simulink model "Log_Optitrack_TruckLab_A1"  (R2025b)
settings: Solver=ode4  StartTime=0  StopTime=130  FixedStep=1/120  RelTol=1e-3
undefined symbols (not defined in the file or in its folder): getRigidBodyPose
libraries: simulink_extras x2
settings Model: Creator=20212285  LastModifiedBy=20224886
settings SolverCC: AlgebraicLoopSolver=LineSearch
settings DataIOCC: ReturnWorkspaceOutputsName=s
settings OptimizationCC: EnhancedBackFolding=on  PassReuseOutputArgsAs=Individual arguments  ZeroExternalMemoryAtStartup=off  ZeroInternalMemoryAtStartup=off  MaxStackSize=64  OptimizeBlockOrder=speed  DifferentSizesBufferReuse=on  OptimizationCustomize=off  EfficientTunableParamExpr=on
settings DebuggingCC: ParameterTunabilityLossMsg=error  UnconnectedInputMsg=warning  UnconnectedOutputMsg=warning  UnconnectedLineMsg=warning
settings ModelReferenceCC: EnableRefExpFcnMdlSchedulingChecks=on
settings SFSimCC: MATLABDynamicMemAlloc=off  SimTargetLang=C++  SimDLTargetLibrary=mkl-dnn
settings RTWCC: SystemTargetFile=ert.tlc  HardwareBoard=Robot Operating System 2 (ROS 2)  TLCOptions="-aInlineSetEventsForThisBaseRateFcn=TLC_FALSE -aSuppressMultiTaskScheduler=TLC_FALSE  -aRateBasedStepFcn=0"  TemplateMakefile=ert_default_tmf  Toolchain=Colcon Tools  TargetLang=C++  GPUComputeCapability=3.5  Description=Embedded Coder
settings CodeAppCC: ForceParamTrailComments=on  IgnoreCustomStorageClasses=off  OperatorAnnotations=on  SimulinkDataObjDesc=on  SFDataObjDesc=on  InsertBlockDesc=on
settings ERTTargetCC: ExtModeTransport=2.0  ExtModeStaticAlloc=on  ExtModeAutomaticAllocSize=off  ExtModeMexFile=ext_xcp  ExtModeIntrfLevel=Level2 - Open  InlinedParameterPlacement=Hierarchical  RootIOFormat=Structure reference  DynamicArrayContainerType=coder::array  CodeInterfacePackaging=C++ class

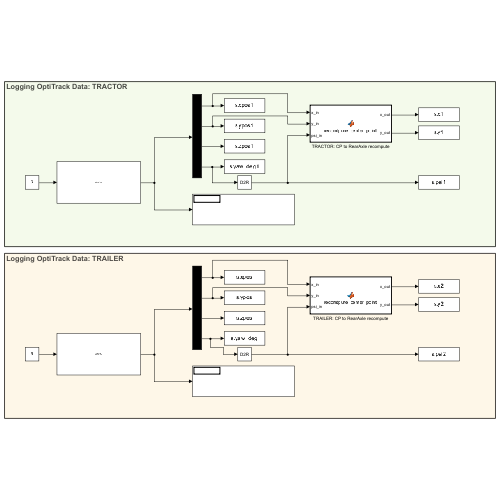
[thumbnail: Simulink's stored preview of the top-level diagram]
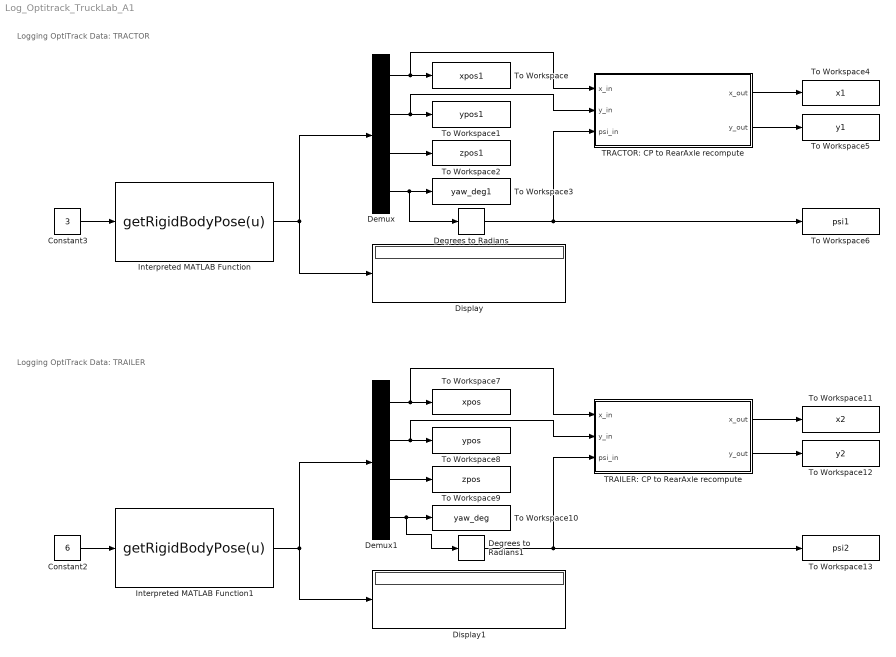
== system Log_Optitrack_TruckLab_A1 ==
  note: Logging OptiTrack Data: TRACTOR
  note: Logging OptiTrack Data: TRAILER
  Constant2 : Constant  Value=6
  Constant3 : Constant  Value=3
  Degrees to Radians : simulink_extras/Transformations/Degrees to Radians
  Degrees to Radians1 : simulink_extras/Transformations/Degrees to Radians
  Demux : Demux
  Demux1 : Demux
  Display : Display
  Display1 : Display
  Interpreted MATLAB Function : MATLABFcn  MATLABFcn=getRigidBodyPose(u)
  Interpreted MATLAB Function1 : MATLABFcn  MATLABFcn=getRigidBodyPose(u)
  TRACTOR: CP to RearAxle recompute : MATLAB Function  TreatAsAtomicUnit=on
  TRAILER: CP to RearAxle recompute : MATLAB Function  TreatAsAtomicUnit=on
  To Workspace : ToWorkspace  VariableName=xpos1  SaveFormat=Timeseries  SampleTime=-1
  To Workspace1 : ToWorkspace  VariableName=ypos1  SaveFormat=Timeseries  SampleTime=-1
  To Workspace10 : ToWorkspace  VariableName=yaw_deg  SaveFormat=Timeseries  SampleTime=-1
  To Workspace11 : ToWorkspace  VariableName=x2  SaveFormat=Timeseries  SampleTime=-1
  To Workspace12 : ToWorkspace  VariableName=y2  SaveFormat=Timeseries  SampleTime=-1
  To Workspace13 : ToWorkspace  VariableName=psi2  SaveFormat=Timeseries  SampleTime=-1
  To Workspace2 : ToWorkspace  VariableName=zpos1  SaveFormat=Timeseries  SampleTime=-1
  To Workspace3 : ToWorkspace  VariableName=yaw_deg1  SaveFormat=Timeseries  SampleTime=-1
  To Workspace4 : ToWorkspace  VariableName=x1  SaveFormat=Timeseries  SampleTime=-1
  To Workspace5 : ToWorkspace  VariableName=y1  SaveFormat=Timeseries  SampleTime=-1
  To Workspace6 : ToWorkspace  VariableName=psi1  SaveFormat=Timeseries  SampleTime=-1
  To Workspace7 : ToWorkspace  VariableName=xpos  SaveFormat=Timeseries  SampleTime=-1
  To Workspace8 : ToWorkspace  VariableName=ypos  SaveFormat=Timeseries  SampleTime=-1
  To Workspace9 : ToWorkspace  VariableName=zpos  SaveFormat=Timeseries  SampleTime=-1
  wires:
  Demux/4 -> Degrees to Radians/1, To Workspace3/1
  Interpreted MATLAB Function/1 -> Display/1, Demux/1
  Demux/1 -> To Workspace/1, TRACTOR: CP to RearAxle recompute/1(x_in)
  Demux/2 -> TRACTOR: CP to RearAxle recompute/2(y_in), To Workspace1/1
  Demux/3 -> To Workspace2/1
  Degrees to Radians/1 -> To Workspace6/1, TRACTOR: CP to RearAxle recompute/3(psi_in)
  TRACTOR: CP to RearAxle recompute/1(x_out) -> To Workspace4/1
  TRACTOR: CP to RearAxle recompute/2(y_out) -> To Workspace5/1
  TRAILER: CP to RearAxle recompute/1(x_out) -> To Workspace11/1
  Degrees to Radians1/1 -> To Workspace13/1, TRAILER: CP to RearAxle recompute/3(psi_in)
  TRAILER: CP to RearAxle recompute/2(y_out) -> To Workspace12/1
  Demux1/1 -> To Workspace7/1, TRAILER: CP to RearAxle recompute/1(x_in)
  Demux1/2 -> TRAILER: CP to RearAxle recompute/2(y_in), To Workspace8/1
  Demux1/4 -> Degrees to Radians1/1, To Workspace10/1
  Demux1/3 -> To Workspace9/1
  Interpreted MATLAB Function1/1 -> Display1/1, Demux1/1
  Constant2/1 -> Interpreted MATLAB Function1/1
  Constant3/1 -> Interpreted MATLAB Function/1

== matlab function Log_Optitrack_TruckLab_A1/TRAILER: CP to RearAxle recompute ==
  data: x_in input; y_in input; psi_in input; x_out output; y_out output
function [x_out, y_out] = recomtpure_center_point(x_in, y_in, psi_in)

    cp_offset = 0.18; %[m]

    x_out = x_in - cp_offset*cos(psi_in);
    y_out = y_in - cp_offset*sin(psi_in);

== matlab function Log_Optitrack_TruckLab_A1/TRACTOR: CP to RearAxle recompute ==
  data: x_in input; y_in input; psi_in input; x_out output; y_out output
function [x_out, y_out] = recomtpure_center_point(x_in, y_in, psi_in)

    cp_offset = 0.31; %[m]

    x_out = x_in - cp_offset*cos(psi_in);
    y_out = y_in - cp_offset*sin(psi_in);
